simulink model "simulink_s2_22b_22c_2020a_03_2"  (R2023b)
settings: Solver=VariableStepAuto  StartTime=0.0  StopTime=10.0  MaxStep=0.001  RelTol=1e-3
values from neighbouring files (symbols this model uses):
  COM = [0 0.001 0.002 0.003 0.004 0.005 0.006 0.007 0.008 0.009 0.01 0.011 ... (30000 elements, 15000x2)]    [kp=4.2-data.mat]    (also in kp=8.7-data.mat; script_s1.m = [time, data(:,2)])
  OUT = [0 0.001 0.002 0.003 0.004 0.005 0.006 0.007 0.008 0.009 0.01 0.011 ... (30000 elements, 15000x2)]    [kp=4.2-data.mat]    (also in kp=8.7-data.mat; script_s1.m = [time, data(:,1)])
  REF = [0 0.001 0.002 0.003 0.004 0.005 0.006 0.007 0.008 0.009 0.01 0.011 ... (30000 elements, 15000x2)]    [kp=4.2-data.mat]    (also in kp=8.7-data.mat)
settings Model: Creator=Admin  LastModifiedBy=lucasp
settings SolverCC: AlgebraicLoopSolver=TrustRegion

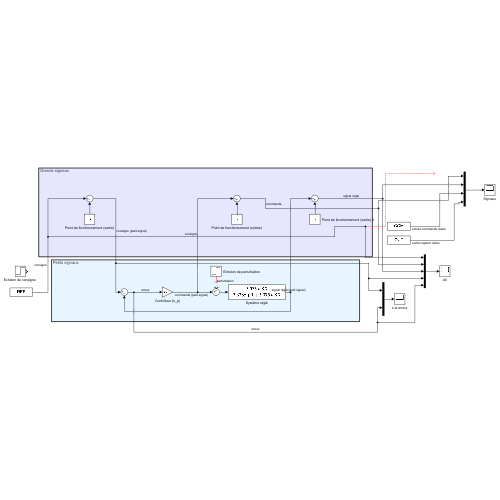
[thumbnail: Simulink's stored preview of the top-level diagram]
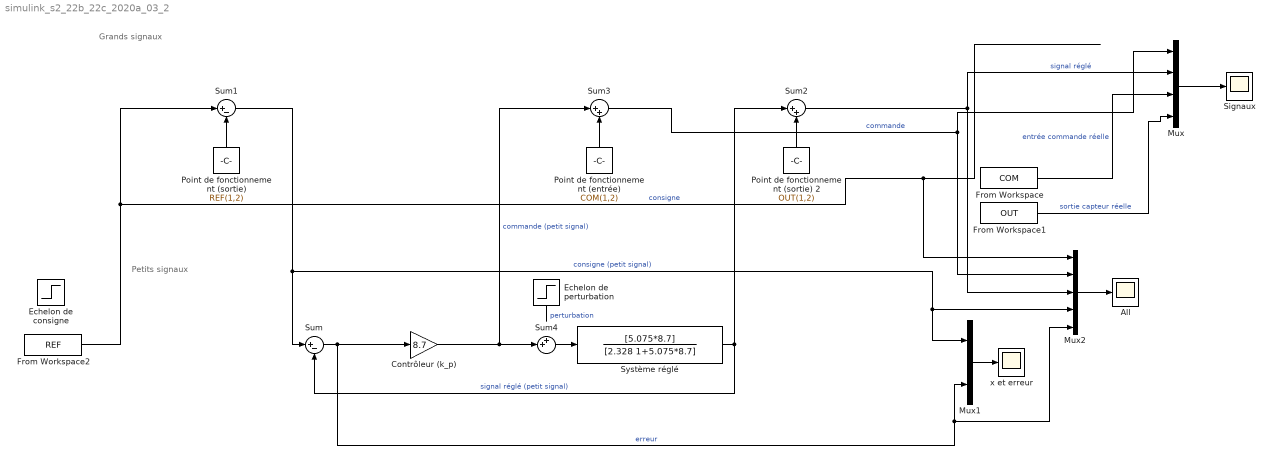
== system simulink_s2_22b_22c_2020a_03_2 ==
  note: Petits signaux
  note: Grands signaux
  All : Scope
  Contrôleur (k_p) : Gain  Gain=8.7
  "Echelon de consigne " : Step  Before=5.782  After=1.5+5.782  SampleTime=0
  Echelon de perturbation : Step  SampleTime=0
  From Workspace : FromWorkspace  VariableName=COM
  From Workspace1 : FromWorkspace  VariableName=OUT
  From Workspace2 : FromWorkspace  VariableName=REF
  Mux : Mux
  Mux1 : Mux  Inputs=2
  Mux2 : Mux  Inputs=5
  Point de fonctionnement (entrée) : Constant  Value=COM(1,2)
  Point de fonctionnement (sortie) : Constant  Value=REF(1,2)
  Point de fonctionnement (sortie) 2 : Constant  Value=OUT(1,2)
  Signaux : Scope
  Sum : Sum  Inputs=|+-
  Sum1 : Sum  Inputs=|+-
  Sum2 : Sum  Inputs=|++
  Sum3 : Sum  Inputs=|++
  Sum4 : Sum  Inputs=++|
  Système réglé : TransferFcn  Numerator=[5.075*8.7]  Denominator=[2.328 1+5.075*8.7]
  x et erreur : Scope
  wires:
  Sum/1 -> Mux2/5, Mux1/2, Contrôleur (k_p)/1  "erreur"
  Contrôleur (k_p)/1 -> Sum4/2, Sum3/1  "commande (petit signal)"
  Système réglé/1 -> Sum/2, Sum2/1  "signal réglé (petit signal)"
  Point de fonctionnement (sortie) 2/1 -> Sum2/2
  Mux/1 -> Signaux/1
  Sum2/1 -> Mux/2, Mux2/3  "signal réglé"
  From Workspace2/1 -> Sum1/1, Mux2/1  "consigne"
  Sum1/1 -> Mux2/4, Mux1/1, Sum/1  "consigne (petit signal)"
  Point de fonctionnement (sortie)/1 -> Sum1/2
  Point de fonctionnement (entrée)/1 -> Sum3/2
  Sum3/1 -> Mux/1, Mux2/2  "commande"
  Sum4/1 -> Système réglé/1
  Echelon de perturbation/1 -> ?  "perturbation"
  Mux1/1 -> x et erreur/1
  Mux2/1 -> All/1
  From Workspace/1 -> Mux/3  "entrée commande réelle"
  From Workspace1/1 -> Mux/4  "sortie capteur réelle"
